simulink library "dc_dc_isolated_converters"  (R2019b)
settings: Solver=VariableStepAuto  StartTime=0.0  StopTime=10.0  RelTol=1e-3
libraries: powerlib x1
settings Model: Creator=mehdi  LastModifiedBy=mehdi

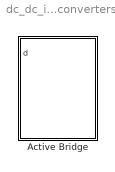
== system dc_dc_isolated_converters ==
  Active Bridge : Subsystem  mask(Active Bridge){f=10e3, adv=off, phase_delay=0, max_delay=10, d_offset=1, start_switching=0}
      mask prompts: f "Switching Frequency (Hz)"; adv "Advance Design"; phase_delay "Default Phase Delay (rad)"; max_delay "MAX Delay Alowed"; d_offset "Phase Shift Offset"; start_switching "Start switching at (sec)"
      mask help:
      | This block designed to accelerat "Multi Active Bridge" simulations with "SPS" switching.
      |
      | Input "d" is phase shift delay in [-1 1].
      |
      | To get more option check "Advance Design".
      mask Callback adv:
      | adv = get_param(gcb, 'adv');
      | mask = Simulink.Mask.get(gcb);
      | pd = mask.getParameter('phase_delay');
      | md = mask.getParameter('max_delay');
      | do = mask.getParameter('d_offset');
      | ss = mask.getParameter('start_switching');
      | 
      | pd.Visible = adv;
      | md.Visible = adv;
      | do.Visible = adv;
      | ss.Visible = adv;
      mask Display: disp('Active\nBridge')

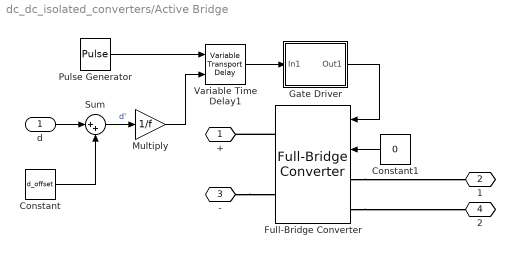
== system dc_dc_isolated_converters/Active Bridge ==
  d : Inport
  Constant : Constant  Value=d_offset
  Constant1 : Constant  Value=0
  Full-Bridge Converter : powerlib/Power Electronics/Full-Bridge Converter  ModelType=Switching devices  Ron=1e-3  Rs=1e6  Cs=inf  Vforward=[0,0]  Ron_Diode=1e-3  Rs_Diode=1e6  Cs_Diode=inf  Vf_Diode=1e-3  Rs_CurrentSource=inf
      settings: SourceProductName=Simscape Electrical  SourceProductBaseCode=PS
  Gate Driver : Subsystem
      mask Display: disp('Gate\nDriver')
  Multiply : Gain  Gain=1/f
  Pulse Generator : DiscretePulseGenerator  PulseType=Time based  Period=1/f  PulseWidth=50  PhaseDelay=phase_delay/(2*pi*f)
  Sum : Sum  Inputs=|++
  Variable Time Delay1 : VariableTransportDelay  MaximumDelay=max_delay
  + : PMIOPort  Side=Left
  1 : PMIOPort  Port=2  Side=Right
  - : PMIOPort  Port=3  Side=Left
  2 : PMIOPort  Port=4  Side=Right
  wires:
  Constant1/1 -> Full-Bridge Converter/2
  Gate Driver/1(Out1) -> Full-Bridge Converter/1
  Sum/1 -> Multiply/1  "d'"
  d/1 -> Sum/1
  Constant/1 -> Sum/2
  Multiply/1 -> Variable Time Delay1/2
  Pulse Generator/1 -> Variable Time Delay1/1
  Variable Time Delay1/1 -> Gate Driver/1(In1)
  connections:
  -/RConn1 -- Full-Bridge Converter/RConn2
  Full-Bridge Converter/LConn1 -- 1/RConn1
  Full-Bridge Converter/LConn2 -- 2/RConn1
  Full-Bridge Converter/RConn1 -- +/RConn1

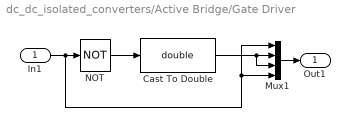
== system dc_dc_isolated_converters/Active Bridge/Gate Driver ==
  In1 : Inport
  Cast To Double : DataTypeConversion  OutDataTypeStr=double
  Mux1 : Mux
  NOT : Logic  Operator=NOT  IconShape=distinctive  AllPortsSameDT=off  OutDataTypeStr=boolean
  Out1 : Outport
  wires:
  Mux1/1 -> Out1/1
  In1/1 -> Mux1/4, Mux1/1, NOT/1
  NOT/1 -> Cast To Double/1
  Cast To Double/1 -> Mux1/3, Mux1/2
